simulink model "mass_sim"  (R2016b)
settings: Solver=ode45  StartTime=0.0  StopTime=100  RelTol=1e-3  EnableMultiTasking=on
InitFcn:
  | loopshape_mass
undefined symbols (not defined in the file or in its folder): mass_ctrl, P
settings Model: Creator=beard  LastModifiedBy=beard
settings DataIOCC: LimitDataPoints=on  SaveFormat=Array  SignalLoggingSaveFormat=ModelDataLogs
settings OptimizationCC: ExpressionDepthLimit=2147483647  InitFltsAndDblsToZero=on  LifeSpan=inf
settings DebuggingCC: UnderspecifiedInitializationDetection=Classic  MergeDetectMultiDrivingBlocksExec=none  SolverPrmCheckMsg=warning  FcnCallInpInsideContextMsg=warning  StateNameClashWarn=warning  SFUnexpectedBacktrackingDiag=warning  SFNoUnconditionalDefaultTransitionDiag=warning  SFExecutionAtInitializationDiag=none
settings HardwareCC: ProdBitPerPointer=32  ProdBitPerSizeT=32  ProdBitPerPtrDiffT=32  ProdLargestAtomicFloat=None  ProdIntDivRoundTo=Undefined  ProdEndianess=Unspecified  ProdWordSize=32  ProdHWDeviceType=32-bit Generic
settings ModelReferenceCC: PropagateSignalLabelsOutOfModel=off
settings GRTTargetCC: TargetLangStandard=C89/C90 (ANSI)  GeneratePreprocessorConditionals=Disable all  CombineOutputUpdateFcns=off  GRTInterface=on
settings ConfigComp: CovMetricSettings=dw  CovHtmlReporting=on  CovSaveCumulativeToWorkspaceVar=on  CovSaveSingleToWorkspaceVar=on  CovExternalEMLEnable=off

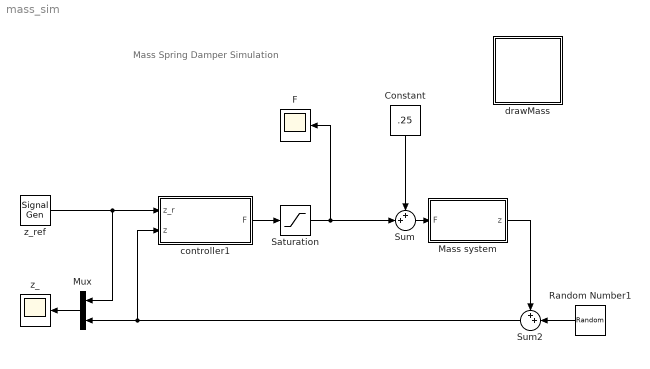
== system mass_sim ==
  note: Mass Spring Damper Simulation
  Constant : Constant  Value=.25
  F : Scope
  Mass system : Subsystem
  Mux : Mux  Inputs=2
  Random Number1 : RandomNumber  Variance=.0001^2  SampleTime=0.1
  Saturation : Saturate  UpperLimit=P.Fmax  LowerLimit=-P.Fmax
  Sum : Sum  Inputs=++|
  Sum2 : Sum  Inputs=++|
  controller1 : Subsystem
  drawMass : Subsystem
      mask Display: image(imread('tv.jpg'))
  z_ : Scope
  z_ref : SignalGenerator  WaveForm=square  Amplitude=.5  Frequency=.02
  wires:
  z_ref/1 -> controller1/1(z_r), Mux/1
  Mux/1 -> z_/1
  controller1/1(F) -> Saturation/1
  Saturation/1 -> Sum/2, F/1
  Sum/1 -> Mass system/1(F)
  Constant/1 -> Sum/1
  Sum2/1 -> controller1/2(z), Mux/2
  Mass system/1(z) -> Sum2/1
  Random Number1/1 -> Sum2/2

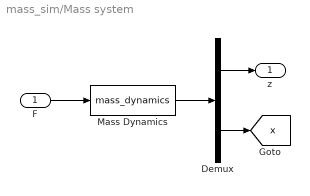
== system mass_sim/Mass system ==
  F : Inport
  Demux : Demux  Outputs=[1;2]
  Mass Dynamics : S-Function  FunctionName=mass_dynamics  Parameters=P  SFunctionDeploymentMode=off  EnableBusSupport=off
  z : Outport
  tag scope: x=global
  wires:
  F/1 -> Mass Dynamics/1
  Mass Dynamics/1 -> Demux/1
  Demux/1 -> z/1
  Demux/2 -> [x]

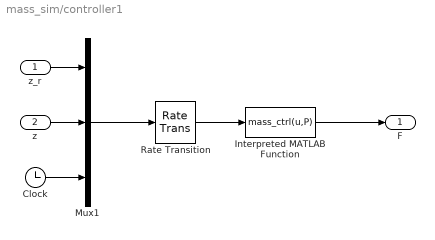
== system mass_sim/controller1 ==
  z_r : Inport
  z : Inport  Port=2
  Clock : Clock
  Interpreted MATLAB Function : MATLABFcn  MATLABFcn=mass_ctrl(u,P)  OutputDimensions=1
  Mux1 : Mux  Inputs=3
  Rate Transition : RateTransition  OutPortSampleTime=P.Ts
  F : Outport
  wires:
  Mux1/1 -> Rate Transition/1
  z_r/1 -> Mux1/1
  z/1 -> Mux1/2
  Clock/1 -> Mux1/3
  Rate Transition/1 -> Interpreted MATLAB Function/1
  Interpreted MATLAB Function/1 -> F/1

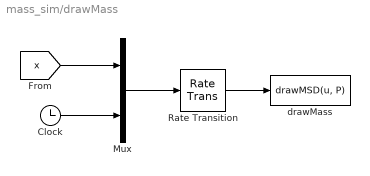
== system mass_sim/drawMass ==
  Clock : Clock
  Mux : Mux  Inputs=2
  Rate Transition : RateTransition  OutPortSampleTime=P.t_plot
  drawMass : MATLABFcn  MATLABFcn=drawMSD(u, P)  OutputDimensions=0
  wires:
  Rate Transition/1 -> drawMass/1
  Clock/1 -> Mux/2
  [x] -> Mux/1
  Mux/1 -> Rate Transition/1
